simulink model "real_plant_A_2014B"  (R2014b)
settings: Solver=ode1  StartTime=0.0  StopTime=sim_run  FixedStep=0.001  RelTol=1e-3
undefined symbols (not defined in the file): AD622, Humusoft, Serial_Port, Standard_Devices, UDP_Protocol, zh_step
libraries: rtwinlib x4
settings Model: CovModelRefEnable=off  CovSFcnEnable=on  Creator=Anony  LastModifiedBy=Anony
settings DataIOCC: SaveFormat=StructureWithTime
settings DebuggingCC: SolverPrmCheckMsg=none  FrameProcessingCompatibilityMsg=error
settings HardwareCC: ProdBitPerPointer=64  ProdLargestAtomicFloat=Float  ProdIntDivRoundTo=Zero  ProdEndianess=LittleEndian  ProdHWDeviceType=Specified
settings GRTTargetCC: GeneratePreprocessorConditionals=Use local settings

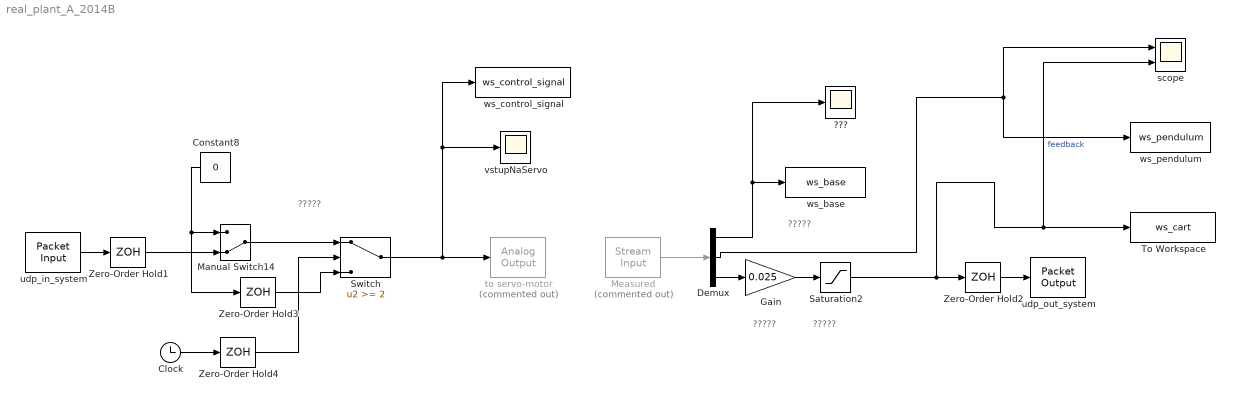
== system real_plant_A_2014B ==
  note: ?????
  note: ?????
  note: ?????
  note: ?????
  "???" : Scope
      settings: TimeRange=10  MaxDataPoints=5000  SaveName=ScopeData2  YMin=170  YMax=222.5  SampleTime=-1
  Clock : Clock
  Constant8 : Constant  Value=0
  Demux : Demux  Outputs=3
  Gain : Gain  Gain=0.025
  Manual Switch14 : ManualSwitch  CurrentSetting=0
  Measured : rtwinlib/Stream Input  Commented=on  SampleTime=0.001  MaxMissedTicks=inf  ShowMissedTicks=off  YieldWhenWaiting=off  DrvName=Standard_Devices/Serial_Port  DrvAddress=1  DrvOptions=[115200 8 0 0 0 0 0 1]  DataTypes='3*double'  FormatString='%f%f%f'  Terminator={'\r\n'}  ShowReady=off  ShowError=off
      settings: AttributesFormatString=Standard Devices\nSerial Port [1h]
  Saturation2 : Saturate  UpperLimit=1650  LowerLimit=25
  Switch : Switch  Threshold=2
  To Workspace : ToWorkspace  VariableName=ws_cart  SaveFormat=Timeseries  SampleTime=-1
  Zero-Order Hold{1..4} (4 alike) : ZeroOrderHold  SampleTime=zh_step
  scope : Scope  NumInputPorts=2
      settings: TimeRange=auto  MaxDataPoints=5000  SaveToWorkspace=off  YMin=-1.00000~15.00000  YMax=1.00000~35.00000  SampleTime=-1
  to servo-motor : rtwinlib/Analog Output  Commented=on  SampleTime=-1  MaxMissedTicks=inf  ShowMissedTicks=off  YieldWhenWaiting=off  DrvName=Humusoft/AD622  DrvAddress=4294967295  DrvOptions=zeros(1,0)  Channels=2  RangeMode=1  VoltRange=1  InitialValue=0  FinalValue=0
      settings: AttributesFormatString=Humusoft\nAD622 [auto]
  udp_in_system : rtwinlib/Packet Input  SampleTime=0.001  MaxMissedTicks=inf  ShowMissedTicks=off  YieldWhenWaiting=off  DrvName=Standard_Devices/UDP_Protocol  DrvAddress=20500  DrvOptions=[2468394756 20500]  PacketSize=8  DataTypes='double'  ShowReady=off  ShowError=off  PacketID=1  ByteOrder=1  ShowTimestamp=off
  udp_out_system : rtwinlib/Packet Output  SampleTime=0.01  MaxMissedTicks=inf  ShowMissedTicks=off  YieldWhenWaiting=off  DrvName=Standard_Devices/UDP_Protocol  DrvAddress=21500  DrvOptions=[2468394756 21500]  PacketSize=8  DataTypes='double'  ShowReady=off  ShowError=off  PacketID=1  ByteOrder=1  InitialValue=[]  FinalValue=[]
  vstupNaServo : Scope
      settings: TimeRange=10  MaxDataPoints=5000  SaveName=ScopeData  YMin=-1.00000  YMax=1.00000  SampleTime=-1
  ws_base : ToWorkspace  VariableName=ws_base  SaveFormat=Timeseries  SampleTime=-1
  ws_control_signal : ToWorkspace  VariableName=ws_control_signal  SaveFormat=Timeseries  SampleTime=-1
  ws_pendulum : ToWorkspace  VariableName=ws_pendulum  SaveFormat=Timeseries  SampleTime=-1
  wires:
  Manual Switch14/1 -> Switch/1
  Switch/1 -> ws_control_signal/1, vstupNaServo/1, to servo-motor/1
  udp_in_system/1 -> Zero-Order Hold1/1
  Demux/3 -> Gain/1
  Measured/1 -> Demux/1
  Gain/1 -> Saturation2/1
  Saturation2/1 -> scope/2, To Workspace/1, Zero-Order Hold2/1  "feedback"
  Demux/2 -> scope/1, ws_pendulum/1
  Demux/1 -> "???"/1, ws_base/1
  Zero-Order Hold1/1 -> Manual Switch14/2
  Zero-Order Hold2/1 -> udp_out_system/1
  Constant8/1 -> Zero-Order Hold3/1, Manual Switch14/1
  Clock/1 -> Zero-Order Hold4/1
  Zero-Order Hold3/1 -> Switch/3
  Zero-Order Hold4/1 -> Switch/2
